simulink model "eCS_Old_Algo_And_Tests"  (R2015b)
settings: Solver=VariableStepAuto  StartTime=0.0  StopTime=10.0  RelTol=1e-3
values from neighbouring files (symbols this model uses):
  pulsetype = 2    [Parameter_eCS_Algo.m]    (also in run_simulation.m = j; run_simulation_ActiveX.m = j)
  rotation = 0    [Parameter_eCS_Algo.m]
  SubPulseType = 1    [Parameter_eCS_Algo.m]
undefined symbols (not defined in the file or in its folder): ddv, DiscIntNeverNeededParam, ECE_45_ax, ECE_45_ay, ECE_45_time, gmw_roada_x__m_s__, gmw_roada_y__m_s__, gmw_roadtime_2kHz, Heiko_AY, Heiko_AY_time, Meldorf_HindenburgstraAcceleration_x__m_s_2_, Meldorf_HindenburgstraAcceleration_y__m_s_2_, Meldorf_HindenburgstraTime__s_, pulse_FF27, pulse_MPDB, pulse_ODB40, pulse_ODB64, pulse_USNCAP, pulsetime_FF27, pulsetime_MPDB, pulsetime_ODB40, pulsetime_ODB64, pulsetime_USNCAP, VW_416_2kHza_x_2kHz, VW_416_2kHza_y_2kHz, VW_416_2kHztime_2kHz
libraries: tllib x9, simulink x9
(part 1 of 8)
settings Model: Creator=pierre-olivier.pilot  LastModifiedBy=pierre-olivier.pilot

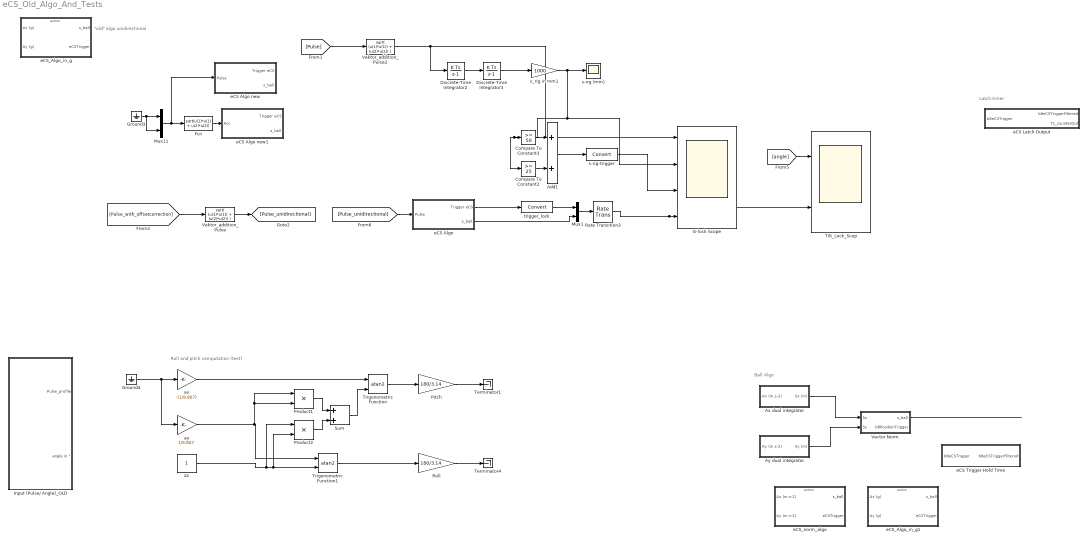
== system eCS_Old_Algo_And_Tests ==
  note: Latch timer
  note: "old" algo unidirectional
  note: Roll and pitch computation (test)
  note: Ball Algo
  Add1 : Sum
  Ax dual integrator : Subsystem  TreatAsAtomicUnit=on
  Ay dual integrator : Subsystem  TreatAsAtomicUnit=on
  Compare To Constant2 : simulink/Logic and Bit Operations/Compare To Constant  relop=>=  const=25  OutDataTypeStr=uint8
  Compare To Constant3 : simulink/Logic and Bit Operations/Compare To Constant  relop=>=  const=50  OutDataTypeStr=uint8
  Discrete-Time Integrator2 : DiscreteIntegrator  InitialConditionSetting=State (most efficient)  SampleTime=-1  ICPrevOutput=DiscIntNeverNeededParam  ICPrevScaledInput=DiscIntNeverNeededParam
  Discrete-Time Integrator3 : DiscreteIntegrator  InitialConditionSetting=State (most efficient)  SampleTime=-1  ICPrevOutput=DiscIntNeverNeededParam  ICPrevScaledInput=DiscIntNeverNeededParam
  Fcn : Fcn  Expr=sqrt(u(1)*u(1) + u(2)*u(2))
  G-lock Scope : Scope  NumInputPorts=4
  Ground3 : Ground
  Ground4 : Ground
  Input (Pulse/ Angle)_OLD : Subsystem
  Mux1 : Mux  Inputs=2
  Mux11 : Mux  Inputs=2
  Pitch : Gain  Gain=180/3.14  mask(TL_Gain){data={'date',738070.39389414352}}
      settings: CopyFcn=if exist('tl_reset_reviewflag') == 2, tl_reset_reviewflag(gcbh); end  DeleteFcn=if exist('delete_tlblock','file')==2,delete_tlblock(gcbh);end  NameChangeFcn=if exist('rename_tlblock','file')==2,rename_tlblock(gcbh);end  OpenFcn=if exist('tl_open_blockdlg','file')==2,tl_open_blockdlg(gcbh);else,open_system(gcbh,'parameter');end
      mask Help: eval(['if exist(''tl_online_help'',''file'') == 2, tl_online_help(''Topic'',''TL_Gain''),else, web([''jar:file:///'',matlabroot,''/help/toolbox/simulink/help.jar!/slref/' lower(get_param(gcbh,'Blocktype')) '.html''], ''-helpbrowser''),end'])
      mask Display: plot([0, .88, 0],[.05, .5, .93]);
  Product1 : Product  Inputs=**  RndMeth=Zero  mask(TL_Product){data={'date',738066.38423623843}}
      settings: CopyFcn=if exist('tl_reset_reviewflag') == 2, tl_reset_reviewflag(gcbh); end  DeleteFcn=if exist('delete_tlblock','file')==2,delete_tlblock(gcbh);end  NameChangeFcn=if exist('rename_tlblock','file')==2,rename_tlblock(gcbh);end  OpenFcn=if exist('tl_open_blockdlg','file')==2,tl_open_blockdlg(gcbh);else,open_system(gcbh,'parameter');end
      mask Help: eval(['if exist(''tl_online_help'',''file'') == 2, tl_online_help(''Topic'',''TL_Product''),else, web([''jar:file:///'',matlabroot,''/help/toolbox/simulink/help.jar!/slref/' lower(get_param(gcbh,'Blocktype')) '.html''], ''-helpbrowser''),end'])
      mask Display: plot([-0.1, 1.05, NaN, -0.1, 1.05],[.01, .01, NaN, .99, .99]);
  Product2 : Product  Inputs=**  RndMeth=Zero  mask(TL_Product){data={'date',738066.38423623843}}
      settings: CopyFcn=if exist('tl_reset_reviewflag') == 2, tl_reset_reviewflag(gcbh); end  DeleteFcn=if exist('delete_tlblock','file')==2,delete_tlblock(gcbh);end  NameChangeFcn=if exist('rename_tlblock','file')==2,rename_tlblock(gcbh);end  OpenFcn=if exist('tl_open_blockdlg','file')==2,tl_open_blockdlg(gcbh);else,open_system(gcbh,'parameter');end
      mask Help: eval(['if exist(''tl_online_help'',''file'') == 2, tl_online_help(''Topic'',''TL_Product''),else, web([''jar:file:///'',matlabroot,''/help/toolbox/simulink/help.jar!/slref/' lower(get_param(gcbh,'Blocktype')) '.html''], ''-helpbrowser''),end'])
      mask Display: plot([-0.1, 1.05, NaN, -0.1, 1.05],[.01, .01, NaN, .99, .99]);
  Rate Transition3 : RateTransition
  Roll : Gain  Gain=180/3.14  mask(TL_Gain){data={'date',738070.3939797685}}
      settings: CopyFcn=if exist('tl_reset_reviewflag') == 2, tl_reset_reviewflag(gcbh); end  DeleteFcn=if exist('delete_tlblock','file')==2,delete_tlblock(gcbh);end  NameChangeFcn=if exist('rename_tlblock','file')==2,rename_tlblock(gcbh);end  OpenFcn=if exist('tl_open_blockdlg','file')==2,tl_open_blockdlg(gcbh);else,open_system(gcbh,'parameter');end
      mask Help: eval(['if exist(''tl_online_help'',''file'') == 2, tl_online_help(''Topic'',''TL_Gain''),else, web([''jar:file:///'',matlabroot,''/help/toolbox/simulink/help.jar!/slref/' lower(get_param(gcbh,'Blocktype')) '.html''], ''-helpbrowser''),end'])
      mask Display: plot([0, .88, 0],[.05, .5, .93]);
  Sum : Sum  mask(TL_Sum){data={'date',738066.38487318286}}
      settings: CopyFcn=if exist('tl_reset_reviewflag') == 2, tl_reset_reviewflag(gcbh); end  DeleteFcn=if exist('delete_tlblock','file')==2,delete_tlblock(gcbh);end  NameChangeFcn=if exist('rename_tlblock','file')==2,rename_tlblock(gcbh);end  OpenFcn=if exist('tl_open_blockdlg','file')==2,tl_open_blockdlg(gcbh);else,open_system(gcbh,'parameter');end
      mask Help: eval(['if exist(''tl_online_help'',''file'') == 2, tl_online_help(''Topic'',''TL_Sum''),else, web([''jar:file:///'',matlabroot,''/help/toolbox/simulink/help.jar!/slref/' lower(get_param(gcbh,'Blocktype')) '.html''], ''-helpbrowser''),end'])
      mask Display: plot([-0.1, 1.05, NaN, -0.1, 1.05],[.01, .01, NaN, .99, .99]);
  Terminator1 : Terminator
  Terminator4 : Terminator
  Tilt_Lock_Scop : Scope  NumInputPorts=2
  Trigonometric Function : Trigonometry  Operator=atan2  mask(TL_Trigonometry){data={'date',738066.38344949076}}
      settings: CopyFcn=if exist('tl_reset_reviewflag') == 2, tl_reset_reviewflag(gcbh); end  DeleteFcn=if exist('delete_tlblock','file')==2,delete_tlblock(gcbh);end  NameChangeFcn=if exist('rename_tlblock','file')==2,rename_tlblock(gcbh);end  OpenFcn=if exist('tl_open_blockdlg','file')==2,tl_open_blockdlg(gcbh);else,open_system(gcbh,'parameter');end
      mask Help: eval(['if exist(''tl_online_help'',''file'') == 2, tl_online_help(''Topic'',''TL_Trigonometry''),else, web([''jar:file:///'',matlabroot,''/help/toolbox/simulink/help.jar!/slref/' lower(get_param(gcbh,'Blocktype')) '.html''], ''-helpbrowser''),end'])
      mask Display: plot([-0.1, 1.05, NaN, -0.1, 1.05],[.01, .01, NaN, .99, .99]);
  Trigonometric Function1 : Trigonometry  Operator=atan2  mask(TL_Trigonometry){data={'date',738066.38344949076}}
      settings: CopyFcn=if exist('tl_reset_reviewflag') == 2, tl_reset_reviewflag(gcbh); end  DeleteFcn=if exist('delete_tlblock','file')==2,delete_tlblock(gcbh);end  NameChangeFcn=if exist('rename_tlblock','file')==2,rename_tlblock(gcbh);end  OpenFcn=if exist('tl_open_blockdlg','file')==2,tl_open_blockdlg(gcbh);else,open_system(gcbh,'parameter');end
      mask Help: eval(['if exist(''tl_online_help'',''file'') == 2, tl_online_help(''Topic'',''TL_Trigonometry''),else, web([''jar:file:///'',matlabroot,''/help/toolbox/simulink/help.jar!/slref/' lower(get_param(gcbh,'Blocktype')) '.html''], ''-helpbrowser''),end'])
      mask Display: plot([-0.1, 1.05, NaN, -0.1, 1.05],[.01, .01, NaN, .99, .99]);
  Vector Norm : Subsystem  TreatAsAtomicUnit=on
  Vektor_addition_Pulse : Fcn  Expr=sqrt( (u(1)*u(1)) + (u(2)*u(2)) )
  Vektor_addition_Pulse2 : Fcn  Expr=sqrt( (u(1)*u(1)) + (u(2)*u(2)) )
  ax : Gain  Gain=-(1/9.807)  mask(TL_Gain){data={'date',738066.38476944447}}
      settings: CopyFcn=if exist('tl_reset_reviewflag') == 2, tl_reset_reviewflag(gcbh); end  DeleteFcn=if exist('delete_tlblock','file')==2,delete_tlblock(gcbh);end  NameChangeFcn=if exist('rename_tlblock','file')==2,rename_tlblock(gcbh);end  OpenFcn=if exist('tl_open_blockdlg','file')==2,tl_open_blockdlg(gcbh);else,open_system(gcbh,'parameter');end
      mask Help: eval(['if exist(''tl_online_help'',''file'') == 2, tl_online_help(''Topic'',''TL_Gain''),else, web([''jar:file:///'',matlabroot,''/help/toolbox/simulink/help.jar!/slref/' lower(get_param(gcbh,'Blocktype')) '.html''], ''-helpbrowser''),end'])
      mask Display: plot([0, .88, 0],[.05, .5, .93]);
  ay : Gain  Gain=1/9.807  mask(TL_Gain){data={'date',738066.375747037}}
      settings: CopyFcn=if exist('tl_reset_reviewflag') == 2, tl_reset_reviewflag(gcbh); end  DeleteFcn=if exist('delete_tlblock','file')==2,delete_tlblock(gcbh);end  NameChangeFcn=if exist('rename_tlblock','file')==2,rename_tlblock(gcbh);end  OpenFcn=if exist('tl_open_blockdlg','file')==2,tl_open_blockdlg(gcbh);else,open_system(gcbh,'parameter');end
      mask Help: eval(['if exist(''tl_online_help'',''file'') == 2, tl_online_help(''Topic'',''TL_Gain''),else, web([''jar:file:///'',matlabroot,''/help/toolbox/simulink/help.jar!/slref/' lower(get_param(gcbh,'Blocktype')) '.html''], ''-helpbrowser''),end'])
      mask Display: plot([0, .88, 0],[.05, .5, .93]);
  az : Constant  mask(TL_Constant){data={'date',738066.3759991898}}
      settings: CopyFcn=if exist('tl_reset_reviewflag') == 2, tl_reset_reviewflag(gcbh); end  DeleteFcn=if exist('delete_tlblock','file')==2,delete_tlblock(gcbh);end  NameChangeFcn=if exist('rename_tlblock','file')==2,rename_tlblock(gcbh);end  OpenFcn=if exist('tl_open_blockdlg','file')==2,tl_open_blockdlg(gcbh);else,open_system(gcbh,'parameter');end
      mask Help: eval(['if exist(''tl_online_help'',''file'') == 2, tl_online_help(''Topic'',''TL_Constant''),else, web([''jar:file:///'',matlabroot,''/help/toolbox/simulink/help.jar!/slref/' lower(get_param(gcbh,'Blocktype')) '.html''], ''-helpbrowser''),end'])
      mask Display: plot([-0.1, 1.05, NaN, -0.1, 1.05],[.01, .01, NaN, .99, .99]);
  eCS Algo : Subsystem
  eCS Algo new : Subsystem
  eCS Algo new1 : Subsystem
  eCS Latch Output : Subsystem  TreatAsAtomicUnit=on
  eCS Trigger Hold Time : Subsystem  TreatAsAtomicUnit=on
  eCS_Algo_in_g : Subsystem
  eCS_Algo_in_g1 : Subsystem
  eCS_norm_algo : Subsystem
  s-rig (mm) : Scope
  s-rig-trigger : DataTypeConversion
  s_rig in mm1 : Gain  Gain=1000
  trigger_lock : DataTypeConversion
  wires:
  Mux1/1 -> Rate Transition3/1
  eCS Algo/1(Trigger eCS) -> trigger_lock/1
  trigger_lock/1 -> Mux1/1
  eCS Algo/2(s_ball) -> Mux1/2
  [angle] -> Tilt_Lock_Scop/1
  Vektor_addition_Pulse/1 -> [Pulse_unidirectional]
  [Pulse_unidirectional] -> eCS Algo/1(Pulse)
  Discrete-Time Integrator2/1 -> Discrete-Time Integrator3/1
  Discrete-Time Integrator3/1 -> s_rig in mm1/1
  Vektor_addition_Pulse2/1 -> Discrete-Time Integrator2/1, G-lock Scope/1
  Compare To Constant2/1 -> Add1/2
  Compare To Constant3/1 -> Add1/1
  s_rig in mm1/1 -> G-lock Scope/2, Compare To Constant2/1, Compare To Constant3/1, s-rig (mm)/1
  Add1/1 -> s-rig-trigger/1
  s-rig-trigger/1 -> G-lock Scope/3
  [Pulse_with_offsetcorrection] -> Vektor_addition_Pulse/1
  [Pulse] -> Vektor_addition_Pulse2/1
  Rate Transition3/1 -> G-lock Scope/4, Tilt_Lock_Scop/2
  Fcn/1 -> eCS Algo new1/1(Acc)
  Mux11/1 -> eCS Algo new/1(Pulse), Fcn/1
  Ground3/1 -> Mux11/2, Mux11/1
  ay/1 -> Product1/2, Product1/1, Trigonometric Function1/1
  az/1 -> Product2/1, Product2/2, Trigonometric Function1/2
  Trigonometric Function1/1 -> Roll/1
  Product1/1 -> Sum/1
  Product2/1 -> Sum/2
  Sum/1 -> Trigonometric Function/2
  Trigonometric Function/1 -> Pitch/1
  Pitch/1 -> Terminator1/1
  Roll/1 -> Terminator4/1
  ax/1 -> Trigonometric Function/1
  Ground4/1 -> ay/1, ax/1
  ? -> Ax dual integrator/1(Ax (m.s-2))
  Vector Norm/1(s_ball) -> ?
  Ax dual integrator/1(Sx (m)) -> Vector Norm/1(Sx)
  Ay dual integrator/1(Sy (m)) -> Vector Norm/2(Sy)
  ? -> Ay dual integrator/1(Ay (m.s-2))

== system eCS_Old_Algo_And_Tests/Ax dual integrator ==
  note: sc: 1e-6
  note: [--64; 63]m.s² => [-32768 ; +32767] LSB
      | scaling : 2^-9
  note: [0 ;25]
  note: [0 ; 25]
  note: Sat [-0.0001 ; 0.0001]g.s²
      | [-10000;10000] LSB
      | scaling : 1e-8
  note: [-2 ; +2] g
      | [-32768 ; 32767] LSB
  note: [-1 : 1]
  note: sc: 1e-6
  note: x-axis : 1e-8
      | y-axis : 1e-4
      | output : 1e-4
  note: sc: 1e-3
  note: sc: 1e-3
  note: sc: 1e-3
  note: sc: 1e-4
  Ax (m.s-2) : Inport
  AddAngle : Sum  mask(TL_Sum){data={'output',{'scaling','PowerOf2/scAngle'},'date',738069.59706952551}}
      settings: CopyFcn=if exist('tl_reset_reviewflag','file')==2,tl_reset_reviewflag(gcbh);end  DeleteFcn=if exist('delete_tlblock','file')==2,delete_tlblock(gcbh);end  NameChangeFcn=if exist('rename_tlblock','file')==2,rename_tlblock(gcbh);end  OpenFcn=if exist('tl_open_blockdlg','file')==2,tl_open_blockdlg(gcbh);else,open_system(gcbh,'parameter');end
      mask Help: eval(['if exist(''tl_online_help'',''file'') == 2, tl_online_help(''Topic'',''TL_Sum''),else, web([''jar:file:///'',matlabroot,''/help/toolbox/simulink/help.jar!/slref/' lower(get_param(gcbh,'Blocktype')) '.html''], ''-helpbrowser''),end'])
      mask Display: plot([-0.1, 1.05, NaN, -0.1, 1.05],[.01, .01, NaN, .99, .99]);
  AddAx : Sum  Inputs=+--  mask(TL_Sum){data={'output',{'type','Int32','scaling','MperSecSqd_Algo/scIntegV_SI'},'date',737961.5188836921}}
      settings: CopyFcn=if exist('tl_reset_reviewflag','file')==2,tl_reset_reviewflag(gcbh);end  DeleteFcn=if exist('delete_tlblock','file')==2,delete_tlblock(gcbh);end  NameChangeFcn=if exist('rename_tlblock','file')==2,rename_tlblock(gcbh);end  OpenFcn=if exist('tl_open_blockdlg','file')==2,tl_open_blockdlg(gcbh);else,open_system(gcbh,'parameter');end
      mask Help: eval(['if exist(''tl_online_help'',''file'') == 2, tl_online_help(''Topic'',''TL_Sum''),else, web([''jar:file:///'',matlabroot,''/help/toolbox/simulink/help.jar!/slref/' lower(get_param(gcbh,'Blocktype')) '.html''], ''-helpbrowser''),end'])
      mask Display: plot([-0.1, 1.05, NaN, -0.1, 1.05],[.01, .01, NaN, .99, .99]);
  AxCalotteAngle1 : Gain  Gain=ddv('eCS_CFG/g_algo/S16_CALOTTE_ANGLE_1')  mask(TL_Gain){data={'output',{'scaling','PowerOf2/scAngle'},'gain',{'variable','eCS_CFG/g_algo/S16_CALOTTE_ANGLE_1'},'date',737958.35980387731}}
      settings: CopyFcn=if exist('tl_reset_reviewflag','file')==2,tl_reset_reviewflag(gcbh);end  DeleteFcn=if exist('delete_tlblock','file')==2,delete_tlblock(gcbh);end  NameChangeFcn=if exist('rename_tlblock','file')==2,rename_tlblock(gcbh);end  OpenFcn=if exist('tl_open_blockdlg','file')==2,tl_open_blockdlg(gcbh);else,open_system(gcbh,'parameter');end
      mask Help: eval(['if exist(''tl_online_help'',''file'') == 2, tl_online_help(''Topic'',''TL_Gain''),else, web([''jar:file:///'',matlabroot,''/help/toolbox/simulink/help.jar!/slref/' lower(get_param(gcbh,'Blocktype')) '.html''], ''-helpbrowser''),end'])
      mask Display: plot([0, .88, 0],[.05, .5, .93]);
  AxCalotteAngle2 : Gain  Gain=ddv('eCS_CFG/g_algo/S16_CALOTTE_ANGLE_2')  mask(TL_Gain){data={'output',{'scaling','PowerOf2/scAngle'},'gain',{'variable','eCS_CFG/g_algo/S16_CALOTTE_ANGLE_2'},'date',737958.35993886576}}
      settings: CopyFcn=if exist('tl_reset_reviewflag','file')==2,tl_reset_reviewflag(gcbh);end  DeleteFcn=if exist('delete_tlblock','file')==2,delete_tlblock(gcbh);end  NameChangeFcn=if exist('rename_tlblock','file')==2,rename_tlblock(gcbh);end  OpenFcn=if exist('tl_open_blockdlg','file')==2,tl_open_blockdlg(gcbh);else,open_system(gcbh,'parameter');end
      mask Help: eval(['if exist(''tl_online_help'',''file'') == 2, tl_online_help(''Topic'',''TL_Gain''),else, web([''jar:file:///'',matlabroot,''/help/toolbox/simulink/help.jar!/slref/' lower(get_param(gcbh,'Blocktype')) '.html''], ''-helpbrowser''),end'])
      mask Display: plot([0, .88, 0],[.05, .5, .93]);
  BallDamperSat : Saturate  UpperLimit=ddv('eCS_CFG/SI_Algo/BALL_DAMPER_SAT_MAX_SI')  LowerLimit=ddv('eCS_CFG/SI_Algo/BALL_DAMPER_SAT_MIN_SI')  mask(TL_Saturate){data={'output',{'type','Int32','scaling','MperSecSqd_Algo/scIntegV_SI'},'lowerlimit',{'variable','eCS_CFG/SI_Algo/BALL_DAMPER_SAT_MIN_SI'},'upperlimit',{'variable','eCS_CFG/SI_Algo/BALL_DAMPER_SAT_MAX_SI'},'date',737957.66559072922}}
      settings: CopyFcn=if exist('tl_reset_reviewflag','file')==2,tl_reset_reviewflag(gcbh);end  DeleteFcn=if exist('delete_tlblock','file')==2,delete_tlblock(gcbh);end  NameChangeFcn=if exist('rename_tlblock','file')==2,rename_tlblock(gcbh);end  OpenFcn=if exist('tl_open_blockdlg','file')==2,tl_open_blockdlg(gcbh);else,open_system(gcbh,'parameter');end
      mask Help: eval(['if exist(''tl_online_help'',''file'') == 2, tl_online_help(''Topic'',''TL_Saturate''),else, web([''jar:file:///'',matlabroot,''/help/toolbox/simulink/help.jar!/slref/' lower(get_param(gcbh,'Blocktype')) '.html''], ''-helpbrowser''),end'])
      mask Display: plot([-0.1, 1.05, NaN, -0.1, 1.05],[.01, .01, NaN, .99, .99]);
  Function : tllib/Function  data={'stepfunctionname','ComputeSx_m','date',737954.54478201387}  displayString=FUNCTION
  IntegSx : DiscreteIntegrator  SampleTime=-1  LimitOutput=on  UpperSaturationLimit=ddv('eCS_CFG/SI_Algo/BALL_POS_MAX_SI')  LowerSaturationLimit=ddv('eCS_CFG/SI_Algo/BALL_POS_MIN_SI')  ICPrevOutput=DiscIntNeverNeededParam  ICPrevScaledInput=DiscIntNeverNeededParam  mask(TL_DiscreteIntegrator){data={'output',{'scaling','MperSecSqd_Algo/scIntegS_SI'},'state',{'scaling','MperSecSqd_Algo/scIntegS_SI'},'lowerlimit',{'variable','eCS_CFG/SI_Algo/BALL_POS_MIN_SI'},'upperlimit',{'variable','eCS_CFG/SI_Algo/BALL_POS_MAX_SI'},'date',738070.37485532404}}
      settings: CopyFcn=if exist('tl_reset_reviewflag') == 2, tl_reset_reviewflag(gcbh); end  DeleteFcn=if exist('delete_tlblock','file')==2,delete_tlblock(gcbh);end  NameChangeFcn=if exist('rename_tlblock','file')==2,rename_tlblock(gcbh);end  OpenFcn=if exist('tl_open_blockdlg','file')==2,tl_open_blockdlg(gcbh);else,open_system(gcbh,'parameter');end
      mask Help: eval(['if exist(''tl_online_help'',''file'') == 2, tl_online_help(''Topic'',''TL_DiscreteIntegrator''),else, web([''jar:file:///'',matlabroot,''/help/toolbox/simulink/help.jar!/slref/' lower(get_param(gcbh,'Blocktype')) '.html''], ''-helpbrowser''),end'])
      mask Display: plot([-0.1, 1.05, NaN, -0.1, 1.05],[.01, .01, NaN, .99, .99]);
  IntegVx : DiscreteIntegrator  SampleTime=-1  ICPrevOutput=DiscIntNeverNeededParam  ICPrevScaledInput=DiscIntNeverNeededParam  mask(TL_DiscreteIntegrator){data={'output',{'scaling','MperSecSqd_Algo/scIntegV_SI'},'state',{'scaling','MperSecSqd_Algo/scIntegV_SI'},'date',737961.51929460652}}
      settings: CopyFcn=if exist('tl_reset_reviewflag') == 2, tl_reset_reviewflag(gcbh); end  DeleteFcn=if exist('delete_tlblock','file')==2,delete_tlblock(gcbh);end  NameChangeFcn=if exist('rename_tlblock','file')==2,rename_tlblock(gcbh);end  OpenFcn=if exist('tl_open_blockdlg','file')==2,tl_open_blockdlg(gcbh);else,open_system(gcbh,'parameter');end
      mask Help: eval(['if exist(''tl_online_help'',''file'') == 2, tl_online_help(''Topic'',''TL_DiscreteIntegrator''),else, web([''jar:file:///'',matlabroot,''/help/toolbox/simulink/help.jar!/slref/' lower(get_param(gcbh,'Blocktype')) '.html''], ''-helpbrowser''),end'])
      mask Display: plot([-0.1, 1.05, NaN, -0.1, 1.05],[.01, .01, NaN, .99, .99]);
  Lut_1_SI : Lookup_n-D  NumberOfTableDimensions=1  BreakpointsForDimension1=ddv('eCS_CFG/SI_Algo/AS8LUT_CALLOTE_ANGLE_1_IDX_SI')  IndexSearchMethod=Linear search  Table=ddv('eCS_CFG/SI_Algo/AS32LUT_CALLOTE_ANGLE_1_FACT_SI')  ExtrapMethod=Clip  UseLastTableValue=on  InternalRulePriority=Speed  RndMeth=Simplest  InputSameDT=on  mask(TL_Lookup1D){data={'input',{'variable','eCS_CFG/SI_Algo/AS8LUT_CALLOTE_ANGLE_1_IDX_SI'},'output',{'scaling','PowerOf2/scLutY'},'table',{'variable','eCS_CFG/SI_Algo/AS32LUT_CALLOTE_ANGLE_1_FACT_SI'},'map',{'name','CalotteAngle1_LUT_SI','class','MERGEABLE_CONST'},'date',737958.39000141202}}
      settings: CopyFcn=if exist('tl_reset_reviewflag','file')==2,tl_reset_reviewflag(gcbh);end  DeleteFcn=if exist('delete_tlblock','file')==2,delete_tlblock(gcbh);end  NameChangeFcn=if exist('rename_tlblock','file')==2,rename_tlblock(gcbh);end  OpenFcn=if exist('tl_open_blockdlg','file')==2,tl_open_blockdlg(gcbh);else,open_system(gcbh,'parameter');end
      mask Help: eval(['if exist(''tl_online_help'',''file'') == 2, tl_online_help(''Topic'',''TL_Lookup1D''),else, web([''jar:file:///'',matlabroot,''/help/toolbox/simulink/help.jar!/slref/' lower(get_param(gcbh,'Blocktype')) '.html''], ''-helpbrowser''),end'])
      mask Display: plot([-0.1, 1.05, NaN, -0.1, 1.05],[.01, .01, NaN, .99, .99]);
  Lut_2_SI : Lookup_n-D  NumberOfTableDimensions=1  BreakpointsForDimension1=ddv('eCS_CFG/SI_Algo/LUT_CALLOTE_ANGLE_2_IDX_SI')  IndexSearchMethod=Linear search  Table=ddv('eCS_CFG/SI_Algo/LUT_CALLOTE_ANGLE_2_FACT_SI')  ExtrapMethod=Clip  UseLastTableValue=on  InternalRulePriority=Speed  RndMeth=Simplest  InputSameDT=on  mask(TL_Lookup1D){data={'input',{'variable','eCS_CFG/SI_Algo/LUT_CALLOTE_ANGLE_2_IDX_SI'},'output',{'scaling','PowerOf2/scLutY'},'table',{'variable','eCS_CFG/SI_Algo/LUT_CALLOTE_ANGLE_2_FACT_SI'},'map',{'name','CalotteAngle2_LUT_SI','class','MERGEABLE_CONST'},'date',737958.39007690968}}
      settings: CopyFcn=if exist('tl_reset_reviewflag','file')==2,tl_reset_reviewflag(gcbh);end  DeleteFcn=if exist('delete_tlblock','file')==2,delete_tlblock(gcbh);end  NameChangeFcn=if exist('rename_tlblock','file')==2,rename_tlblock(gcbh);end  OpenFcn=if exist('tl_open_blockdlg','file')==2,tl_open_blockdlg(gcbh);else,open_system(gcbh,'parameter');end
      mask Help: eval(['if exist(''tl_online_help'',''file'') == 2, tl_online_help(''Topic'',''TL_Lookup1D''),else, web([''jar:file:///'',matlabroot,''/help/toolbox/simulink/help.jar!/slref/' lower(get_param(gcbh,'Blocktype')) '.html''], ''-helpbrowser''),end'])
      mask Display: plot([-0.1, 1.05, NaN, -0.1, 1.05],[.01, .01, NaN, .99, .99]);
  Scope1 : Scope
  SinAx : Trigonometry  mask(TL_Trigonometry){data={'output',{'scaling','PowerOf2/scRadian'},'date',738070.42230274307}}
      settings: CopyFcn=if exist('tl_reset_reviewflag','file')==2,tl_reset_reviewflag(gcbh);end  DeleteFcn=if exist('delete_tlblock','file')==2,delete_tlblock(gcbh);end  NameChangeFcn=if exist('rename_tlblock','file')==2,rename_tlblock(gcbh);end  OpenFcn=if exist('tl_open_blockdlg','file')==2,tl_open_blockdlg(gcbh);else,open_system(gcbh,'parameter');end
      mask Help: eval(['if exist(''tl_online_help'',''file'') == 2, tl_online_help(''Topic'',''TL_Trigonometry''),else, web([''jar:file:///'',matlabroot,''/help/toolbox/simulink/help.jar!/slref/' lower(get_param(gcbh,'Blocktype')) '.html''], ''-helpbrowser''),end'])
      mask Display: plot([-0.1, 1.05, NaN, -0.1, 1.05],[.01, .01, NaN, .99, .99]);
  ball damper : Gain  Gain=ddv('eCS_CFG/g_algo/BALL_DAMPER_COEFF')  mask(TL_Gain){data={'output',{'type','Int32','scaling','MperSecSqd_Algo/scIntegV_SI'},'gain',{'variable','eCS_CFG/g_algo/BALL_DAMPER_COEFF'},'date',737958.37810400466}}
      settings: CopyFcn=if exist('tl_reset_reviewflag','file')==2,tl_reset_reviewflag(gcbh);end  DeleteFcn=if exist('delete_tlblock','file')==2,delete_tlblock(gcbh);end  NameChangeFcn=if exist('rename_tlblock','file')==2,rename_tlblock(gcbh);end  OpenFcn=if exist('tl_open_blockdlg','file')==2,tl_open_blockdlg(gcbh);else,open_system(gcbh,'parameter');end
      mask Help: eval(['if exist(''tl_online_help'',''file'') == 2, tl_online_help(''Topic'',''TL_Gain''),else, web([''jar:file:///'',matlabroot,''/help/toolbox/simulink/help.jar!/slref/' lower(get_param(gcbh,'Blocktype')) '.html''], ''-helpbrowser''),end'])
      mask Display: plot([0, .88, 0],[.05, .5, .93]);
  g to m.s² : Gain  Gain=9.807  mask(TL_Gain){data={'logdata',{'loggingmode',1},'output',{'scaling','MperSecSqd_Algo/scAccel_SI'},'date',738036.70470343751}}
      settings: CopyFcn=if exist('tl_reset_reviewflag','file')==2,tl_reset_reviewflag(gcbh);end  DeleteFcn=if exist('delete_tlblock','file')==2,delete_tlblock(gcbh);end  NameChangeFcn=if exist('rename_tlblock','file')==2,rename_tlblock(gcbh);end  OpenFcn=if exist('tl_open_blockdlg','file')==2,tl_open_blockdlg(gcbh);else,open_system(gcbh,'parameter');end
      mask Help: eval(['if exist(''tl_online_help'',''file'') == 2, tl_online_help(''Topic'',''TL_Gain''),else, web([''jar:file:///'',matlabroot,''/help/toolbox/simulink/help.jar!/slref/' lower(get_param(gcbh,'Blocktype')) '.html''], ''-helpbrowser''),end'])
      mask Display: plot([0, .88, 0],[.05, .5, .93]);
  grad in rad1 : Gain  Gain=pi/180  mask(TL_Gain){data={'output',{'scaling','PowerOf2/scLutY'},'date',737951.6866806366}}
      settings: CopyFcn=if exist('tl_reset_reviewflag','file')==2,tl_reset_reviewflag(gcbh);end  DeleteFcn=if exist('delete_tlblock','file')==2,delete_tlblock(gcbh);end  NameChangeFcn=if exist('rename_tlblock','file')==2,rename_tlblock(gcbh);end  OpenFcn=if exist('tl_open_blockdlg','file')==2,tl_open_blockdlg(gcbh);else,open_system(gcbh,'parameter');end
      mask Help: eval(['if exist(''tl_online_help'',''file'') == 2, tl_online_help(''Topic'',''TL_Gain''),else, web([''jar:file:///'',matlabroot,''/help/toolbox/simulink/help.jar!/slref/' lower(get_param(gcbh,'Blocktype')) '.html''], ''-helpbrowser''),end'])
      mask Display: plot([0, .88, 0],[.05, .5, .93]);
  Sx (m) : Outport
  wires:
  IntegSx/1 -> Sx (m)/1, Lut_1_SI/1, Lut_2_SI/1
  ball damper/1 -> BallDamperSat/1
  AddAngle/1 -> grad in rad1/1
  AxCalotteAngle2/1 -> AddAngle/2
  Lut_2_SI/1 -> AxCalotteAngle2/1
  AxCalotteAngle1/1 -> AddAngle/1
  Lut_1_SI/1 -> AxCalotteAngle1/1
  grad in rad1/1 -> SinAx/1
  BallDamperSat/1 -> AddAx/3
  IntegVx/1 -> IntegSx/1, ball damper/1
  Ax (m.s-2)/1 -> AddAx/1
  AddAx/1 -> Scope1/1, IntegVx/1  "a-ref"
  SinAx/1 -> g to m.s²/1
  g to m.s²/1 -> AddAx/2

== system eCS_Old_Algo_And_Tests/Ay dual integrator ==
  note: sc: 1e-4
  note: sc: 1e-3
  note: sc: 1e-3
  note: sc: 1e-3
  note: x-axis : 1e-8
      | y-axis : 1e-4
      | output : 1e-4
  note: sc: 1e-6
  note: [-1 : 1]
  note: [-2 ; +2] g
      | [-32768 ; 32767] LSB
  note: Sat [-0.0001 ; 0.0001]g.s²
      | [-10000;10000] LSB
      | scaling : 1e-8
  note: [0 ; 25]
  note: [0 ;25]
  note: [--64; 63]m.s² => [-32768 ; +32767] LSB
      | scaling : 2^-9
  note: sc: 1e-6
  Ay (m.s-2) : Inport
  AddAngle : Sum  mask(TL_Sum){data={'output',{'scaling','PowerOf2/scAngle'},'date',737951.68910436344}}
      settings: CopyFcn=if exist('tl_reset_reviewflag','file')==2,tl_reset_reviewflag(gcbh);end  DeleteFcn=if exist('delete_tlblock','file')==2,delete_tlblock(gcbh);end  NameChangeFcn=if exist('rename_tlblock','file')==2,rename_tlblock(gcbh);end  OpenFcn=if exist('tl_open_blockdlg','file')==2,tl_open_blockdlg(gcbh);else,open_system(gcbh,'parameter');end
      mask Help: eval(['if exist(''tl_online_help'',''file'') == 2, tl_online_help(''Topic'',''TL_Sum''),else, web([''jar:file:///'',matlabroot,''/help/toolbox/simulink/help.jar!/slref/' lower(get_param(gcbh,'Blocktype')) '.html''], ''-helpbrowser''),end'])
      mask Display: plot([-0.1, 1.05, NaN, -0.1, 1.05],[.01, .01, NaN, .99, .99]);
  AddAy : Sum  Inputs=+--  mask(TL_Sum){data={'output',{'type','Int32','scaling','MperSecSqd_Algo/scIntegV_SI'},'date',738036.68940328702}}
      settings: CopyFcn=if exist('tl_reset_reviewflag','file')==2,tl_reset_reviewflag(gcbh);end  DeleteFcn=if exist('delete_tlblock','file')==2,delete_tlblock(gcbh);end  NameChangeFcn=if exist('rename_tlblock','file')==2,rename_tlblock(gcbh);end  OpenFcn=if exist('tl_open_blockdlg','file')==2,tl_open_blockdlg(gcbh);else,open_system(gcbh,'parameter');end
      mask Help: eval(['if exist(''tl_online_help'',''file'') == 2, tl_online_help(''Topic'',''TL_Sum''),else, web([''jar:file:///'',matlabroot,''/help/toolbox/simulink/help.jar!/slref/' lower(get_param(gcbh,'Blocktype')) '.html''], ''-helpbrowser''),end'])
      mask Display: plot([-0.1, 1.05, NaN, -0.1, 1.05],[.01, .01, NaN, .99, .99]);
  AyCalotteAngle1 : Gain  Gain=ddv('eCS_CFG/g_algo/S16_CALOTTE_ANGLE_1')  mask(TL_Gain){data={'output',{'scaling','PowerOf2/scAngle'},'gain',{'variable','eCS_CFG/g_algo/S16_CALOTTE_ANGLE_1'},'date',737958.36027694447}}
      settings: CopyFcn=if exist('tl_reset_reviewflag','file')==2,tl_reset_reviewflag(gcbh);end  DeleteFcn=if exist('delete_tlblock','file')==2,delete_tlblock(gcbh);end  NameChangeFcn=if exist('rename_tlblock','file')==2,rename_tlblock(gcbh);end  OpenFcn=if exist('tl_open_blockdlg','file')==2,tl_open_blockdlg(gcbh);else,open_system(gcbh,'parameter');end
      mask Help: eval(['if exist(''tl_online_help'',''file'') == 2, tl_online_help(''Topic'',''TL_Gain''),else, web([''jar:file:///'',matlabroot,''/help/toolbox/simulink/help.jar!/slref/' lower(get_param(gcbh,'Blocktype')) '.html''], ''-helpbrowser''),end'])
      mask Display: plot([0, .88, 0],[.05, .5, .93]);
  AyCalotteAngle2 : Gain  Gain=ddv('eCS_CFG/g_algo/S16_CALOTTE_ANGLE_2')  mask(TL_Gain){data={'output',{'scaling','PowerOf2/scAngle'},'gain',{'variable','eCS_CFG/g_algo/S16_CALOTTE_ANGLE_2'},'date',737958.36034565978}}
      settings: CopyFcn=if exist('tl_reset_reviewflag','file')==2,tl_reset_reviewflag(gcbh);end  DeleteFcn=if exist('delete_tlblock','file')==2,delete_tlblock(gcbh);end  NameChangeFcn=if exist('rename_tlblock','file')==2,rename_tlblock(gcbh);end  OpenFcn=if exist('tl_open_blockdlg','file')==2,tl_open_blockdlg(gcbh);else,open_system(gcbh,'parameter');end
      mask Help: eval(['if exist(''tl_online_help'',''file'') == 2, tl_online_help(''Topic'',''TL_Gain''),else, web([''jar:file:///'',matlabroot,''/help/toolbox/simulink/help.jar!/slref/' lower(get_param(gcbh,'Blocktype')) '.html''], ''-helpbrowser''),end'])
      mask Display: plot([0, .88, 0],[.05, .5, .93]);
  BallDamperSat : Saturate  UpperLimit=ddv('eCS_CFG/SI_Algo/BALL_DAMPER_SAT_MAX_SI')  LowerLimit=ddv('eCS_CFG/SI_Algo/BALL_DAMPER_SAT_MIN_SI')  mask(TL_Saturate){data={'output',{'type','Int32','scaling','MperSecSqd_Algo/scIntegV_SI'},'lowerlimit',{'variable','eCS_CFG/SI_Algo/BALL_DAMPER_SAT_MIN_SI'},'upperlimit',{'variable','eCS_CFG/SI_Algo/BALL_DAMPER_SAT_MAX_SI'},'date',737957.66570109956}}
      settings: CopyFcn=if exist('tl_reset_reviewflag','file')==2,tl_reset_reviewflag(gcbh);end  DeleteFcn=if exist('delete_tlblock','file')==2,delete_tlblock(gcbh);end  NameChangeFcn=if exist('rename_tlblock','file')==2,rename_tlblock(gcbh);end  OpenFcn=if exist('tl_open_blockdlg','file')==2,tl_open_blockdlg(gcbh);else,open_system(gcbh,'parameter');end
      mask Help: eval(['if exist(''tl_online_help'',''file'') == 2, tl_online_help(''Topic'',''TL_Saturate''),else, web([''jar:file:///'',matlabroot,''/help/toolbox/simulink/help.jar!/slref/' lower(get_param(gcbh,'Blocktype')) '.html''], ''-helpbrowser''),end'])
      mask Display: plot([-0.1, 1.05, NaN, -0.1, 1.05],[.01, .01, NaN, .99, .99]);
  Function : tllib/Function  data={'stepfunctionname','ComputeSy_m','date',737957.66316383099}  displayString=FUNCTION
  IntegSy : DiscreteIntegrator  SampleTime=-1  LimitOutput=on  UpperSaturationLimit=ddv('eCS_CFG/SI_Algo/BALL_POS_MAX_SI')  LowerSaturationLimit=ddv('eCS_CFG/SI_Algo/BALL_POS_MIN_SI')  ICPrevOutput=DiscIntNeverNeededParam  ICPrevScaledInput=DiscIntNeverNeededParam  mask(TL_DiscreteIntegrator){data={'output',{'scaling','MperSecSqd_Algo/scIntegS_SI'},'state',{'scaling','MperSecSqd_Algo/scIntegS_SI'},'lowerlimit',{'variable','eCS_CFG/SI_Algo/BALL_POS_MIN_SI'},'upperlimit',{'variable','eCS_CFG/SI_Algo/BALL_POS_MAX_SI'},'date',738070.37508417829}}
      settings: CopyFcn=if exist('tl_reset_reviewflag') == 2, tl_reset_reviewflag(gcbh); end  DeleteFcn=if exist('delete_tlblock','file')==2,delete_tlblock(gcbh);end  NameChangeFcn=if exist('rename_tlblock','file')==2,rename_tlblock(gcbh);end  OpenFcn=if exist('tl_open_blockdlg','file')==2,tl_open_blockdlg(gcbh);else,open_system(gcbh,'parameter');end
      mask Help: eval(['if exist(''tl_online_help'',''file'') == 2, tl_online_help(''Topic'',''TL_DiscreteIntegrator''),else, web([''jar:file:///'',matlabroot,''/help/toolbox/simulink/help.jar!/slref/' lower(get_param(gcbh,'Blocktype')) '.html''], ''-helpbrowser''),end'])
      mask Display: plot([-0.1, 1.05, NaN, -0.1, 1.05],[.01, .01, NaN, .99, .99]);
  IntegVy : DiscreteIntegrator  SampleTime=-1  ICPrevOutput=DiscIntNeverNeededParam  ICPrevScaledInput=DiscIntNeverNeededParam  mask(TL_DiscreteIntegrator){data={'output',{'scaling','MperSecSqd_Algo/scIntegV_SI'},'state',{'scaling','MperSecSqd_Algo/scIntegV_SI'},'date',737961.52197425929}}
      settings: CopyFcn=if exist('tl_reset_reviewflag') == 2, tl_reset_reviewflag(gcbh); end  DeleteFcn=if exist('delete_tlblock','file')==2,delete_tlblock(gcbh);end  NameChangeFcn=if exist('rename_tlblock','file')==2,rename_tlblock(gcbh);end  OpenFcn=if exist('tl_open_blockdlg','file')==2,tl_open_blockdlg(gcbh);else,open_system(gcbh,'parameter');end
      mask Help: eval(['if exist(''tl_online_help'',''file'') == 2, tl_online_help(''Topic'',''TL_DiscreteIntegrator''),else, web([''jar:file:///'',matlabroot,''/help/toolbox/simulink/help.jar!/slref/' lower(get_param(gcbh,'Blocktype')) '.html''], ''-helpbrowser''),end'])
      mask Display: plot([-0.1, 1.05, NaN, -0.1, 1.05],[.01, .01, NaN, .99, .99]);
  Lut_1_SI : Lookup_n-D  NumberOfTableDimensions=1  BreakpointsForDimension1=ddv('eCS_CFG/SI_Algo/AS8LUT_CALLOTE_ANGLE_1_IDX_SI')  IndexSearchMethod=Linear search  Table=ddv('eCS_CFG/SI_Algo/AS32LUT_CALLOTE_ANGLE_1_FACT_SI')  ExtrapMethod=Clip  UseLastTableValue=on  InternalRulePriority=Speed  RndMeth=Simplest  InputSameDT=on  mask(TL_Lookup1D){data={'input',{'variable','eCS_CFG/SI_Algo/AS8LUT_CALLOTE_ANGLE_1_IDX_SI'},'output',{'scaling','PowerOf2/scLutY'},'table',{'variable','eCS_CFG/SI_Algo/AS32LUT_CALLOTE_ANGLE_1_FACT_SI'},'map',{'name','CalotteAngle1_LUT_SI','class','MERGEABLE_CONST'},'date',737958.39018503472}}
      settings: CopyFcn=if exist('tl_reset_reviewflag','file')==2,tl_reset_reviewflag(gcbh);end  DeleteFcn=if exist('delete_tlblock','file')==2,delete_tlblock(gcbh);end  NameChangeFcn=if exist('rename_tlblock','file')==2,rename_tlblock(gcbh);end  OpenFcn=if exist('tl_open_blockdlg','file')==2,tl_open_blockdlg(gcbh);else,open_system(gcbh,'parameter');end
      mask Help: eval(['if exist(''tl_online_help'',''file'') == 2, tl_online_help(''Topic'',''TL_Lookup1D''),else, web([''jar:file:///'',matlabroot,''/help/toolbox/simulink/help.jar!/slref/' lower(get_param(gcbh,'Blocktype')) '.html''], ''-helpbrowser''),end'])
      mask Display: plot([-0.1, 1.05, NaN, -0.1, 1.05],[.01, .01, NaN, .99, .99]);
  Lut_2_SI : Lookup_n-D  NumberOfTableDimensions=1  BreakpointsForDimension1=ddv('eCS_CFG/SI_Algo/LUT_CALLOTE_ANGLE_2_IDX_SI')  IndexSearchMethod=Linear search  Table=ddv('eCS_CFG/SI_Algo/LUT_CALLOTE_ANGLE_2_FACT_SI')  ExtrapMethod=Clip  UseLastTableValue=on  InternalRulePriority=Speed  RndMeth=Simplest  InputSameDT=on  mask(TL_Lookup1D){data={'input',{'variable','eCS_CFG/SI_Algo/LUT_CALLOTE_ANGLE_2_IDX_SI'},'output',{'scaling','PowerOf2/scLutY'},'table',{'variable','eCS_CFG/SI_Algo/LUT_CALLOTE_ANGLE_2_FACT_SI'},'map',{'name','CalotteAngle2_LUT_SI','class','MERGEABLE_CONST'},'date',737958.39026763884}}
      settings: CopyFcn=if exist('tl_reset_reviewflag','file')==2,tl_reset_reviewflag(gcbh);end  DeleteFcn=if exist('delete_tlblock','file')==2,delete_tlblock(gcbh);end  NameChangeFcn=if exist('rename_tlblock','file')==2,rename_tlblock(gcbh);end  OpenFcn=if exist('tl_open_blockdlg','file')==2,tl_open_blockdlg(gcbh);else,open_system(gcbh,'parameter');end
      mask Help: eval(['if exist(''tl_online_help'',''file'') == 2, tl_online_help(''Topic'',''TL_Lookup1D''),else, web([''jar:file:///'',matlabroot,''/help/toolbox/simulink/help.jar!/slref/' lower(get_param(gcbh,'Blocktype')) '.html''], ''-helpbrowser''),end'])
      mask Display: plot([-0.1, 1.05, NaN, -0.1, 1.05],[.01, .01, NaN, .99, .99]);
  Scope1 : Scope
  SinAy : Trigonometry  mask(TL_Trigonometry){data={'output',{'scaling','PowerOf2/scRadian'},'date',738036.69720550929}}
      settings: CopyFcn=if exist('tl_reset_reviewflag','file')==2,tl_reset_reviewflag(gcbh);end  DeleteFcn=if exist('delete_tlblock','file')==2,delete_tlblock(gcbh);end  NameChangeFcn=if exist('rename_tlblock','file')==2,rename_tlblock(gcbh);end  OpenFcn=if exist('tl_open_blockdlg','file')==2,tl_open_blockdlg(gcbh);else,open_system(gcbh,'parameter');end
      mask Help: eval(['if exist(''tl_online_help'',''file'') == 2, tl_online_help(''Topic'',''TL_Trigonometry''),else, web([''jar:file:///'',matlabroot,''/help/toolbox/simulink/help.jar!/slref/' lower(get_param(gcbh,'Blocktype')) '.html''], ''-helpbrowser''),end'])
      mask Display: plot([-0.1, 1.05, NaN, -0.1, 1.05],[.01, .01, NaN, .99, .99]);
  ball damper : Gain  Gain=ddv('eCS_CFG/g_algo/BALL_DAMPER_COEFF')  mask(TL_Gain){data={'output',{'type','Int32','scaling','MperSecSqd_Algo/scIntegV_SI'},'gain',{'variable','eCS_CFG/g_algo/BALL_DAMPER_COEFF'},'date',737954.48961925926}}
      settings: CopyFcn=if exist('tl_reset_reviewflag','file')==2,tl_reset_reviewflag(gcbh);end  DeleteFcn=if exist('delete_tlblock','file')==2,delete_tlblock(gcbh);end  NameChangeFcn=if exist('rename_tlblock','file')==2,rename_tlblock(gcbh);end  OpenFcn=if exist('tl_open_blockdlg','file')==2,tl_open_blockdlg(gcbh);else,open_system(gcbh,'parameter');end
      mask Help: eval(['if exist(''tl_online_help'',''file'') == 2, tl_online_help(''Topic'',''TL_Gain''),else, web([''jar:file:///'',matlabroot,''/help/toolbox/simulink/help.jar!/slref/' lower(get_param(gcbh,'Blocktype')) '.html''], ''-helpbrowser''),end'])
      mask Display: plot([0, .88, 0],[.05, .5, .93]);
  g to m.s² : Gain  Gain=9.807  mask(TL_Gain){data={'output',{'scaling','MperSecSqd_Algo/scAccel_SI'},'date',738070.42273535882}}
      settings: CopyFcn=if exist('tl_reset_reviewflag','file')==2,tl_reset_reviewflag(gcbh);end  DeleteFcn=if exist('delete_tlblock','file')==2,delete_tlblock(gcbh);end  NameChangeFcn=if exist('rename_tlblock','file')==2,rename_tlblock(gcbh);end  OpenFcn=if exist('tl_open_blockdlg','file')==2,tl_open_blockdlg(gcbh);else,open_system(gcbh,'parameter');end
      mask Help: eval(['if exist(''tl_online_help'',''file'') == 2, tl_online_help(''Topic'',''TL_Gain''),else, web([''jar:file:///'',matlabroot,''/help/toolbox/simulink/help.jar!/slref/' lower(get_param(gcbh,'Blocktype')) '.html''], ''-helpbrowser''),end'])
      mask Display: plot([0, .88, 0],[.05, .5, .93]);
  grad in rad1 : Gain  Gain=pi/180  mask(TL_Gain){data={'output',{'scaling','PowerOf2/scLutY'},'date',737951.6866806366}}
      settings: CopyFcn=if exist('tl_reset_reviewflag','file')==2,tl_reset_reviewflag(gcbh);end  DeleteFcn=if exist('delete_tlblock','file')==2,delete_tlblock(gcbh);end  NameChangeFcn=if exist('rename_tlblock','file')==2,rename_tlblock(gcbh);end  OpenFcn=if exist('tl_open_blockdlg','file')==2,tl_open_blockdlg(gcbh);else,open_system(gcbh,'parameter');end
      mask Help: eval(['if exist(''tl_online_help'',''file'') == 2, tl_online_help(''Topic'',''TL_Gain''),else, web([''jar:file:///'',matlabroot,''/help/toolbox/simulink/help.jar!/slref/' lower(get_param(gcbh,'Blocktype')) '.html''], ''-helpbrowser''),end'])
      mask Display: plot([0, .88, 0],[.05, .5, .93]);
  Sy (m) : Outport
  wires:
  g to m.s²/1 -> AddAy/2
  SinAy/1 -> g to m.s²/1
  AddAy/1 -> IntegVy/1, Scope1/1  "a-ref"
  Ay (m.s-2)/1 -> AddAy/1
  IntegVy/1 -> ball damper/1, IntegSy/1
  BallDamperSat/1 -> AddAy/3
  grad in rad1/1 -> SinAy/1
  Lut_1_SI/1 -> AyCalotteAngle1/1
  AyCalotteAngle1/1 -> AddAngle/1
  Lut_2_SI/1 -> AyCalotteAngle2/1
  AyCalotteAngle2/1 -> AddAngle/2
  AddAngle/1 -> grad in rad1/1
  ball damper/1 -> BallDamperSat/1
  IntegSy/1 -> Lut_2_SI/1, Lut_1_SI/1, Sy (m)/1

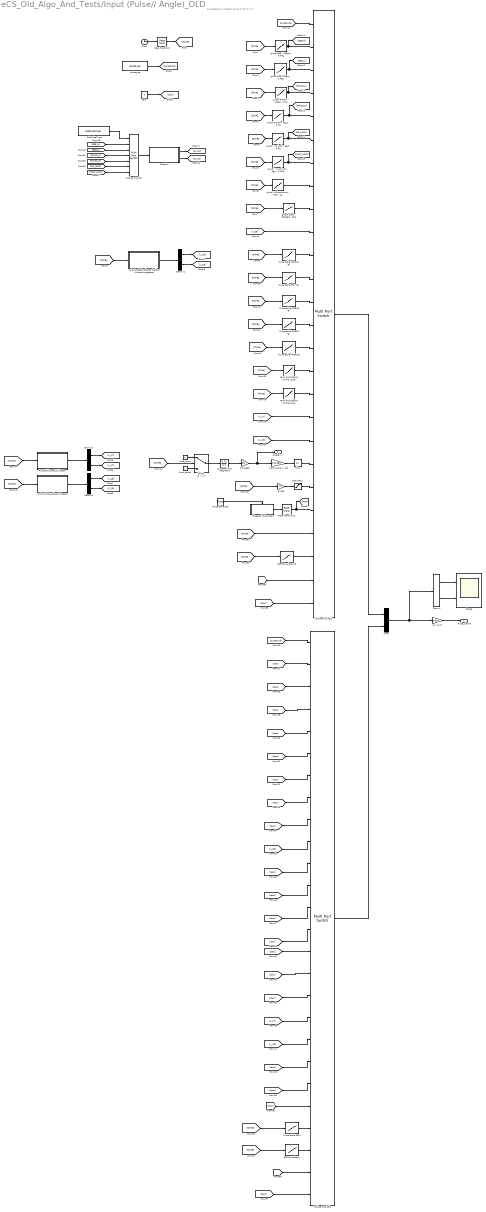
== system eCS_Old_Algo_And_Tests/Input (Pulse// Angle)_OLD ==
  note: pulse tables must begin and end with 0 !!!!!!!
  BMW QV72003-3 no-fire lower : Lookup_n-D  NumberOfTableDimensions=1  BreakpointsForDimension1=[-0.011 0.00 0.020 0.045 0.059]  Table=[0 0 11.0 11.0 0]  ExtrapMethod=Clip  UseLastTableValue=on  InternalRulePriority=Speed  RndMeth=Simplest  InputSameDT=on
  BMW QV72003-3 no-fire upper : Lookup_n-D  NumberOfTableDimensions=1  BreakpointsForDimension1=[0 0.027 0.059 0.085]  Table=[0 16.2 16.2 0]  ExtrapMethod=Clip  UseLastTableValue=on  InternalRulePriority=Speed  RndMeth=Simplest  InputSameDT=on
  Clock : Clock
  Demux{,1..3} (4 alike) : Demux  Outputs=2
  Discrete-Time Integrator4 : DiscreteIntegrator  gainval=1  InitialConditionSetting=State (most efficient)  SampleTime=-1  UpperSaturationLimit=0.3 * 9.81  LowerSaturationLimit=-0.3 * 9.81  ICPrevOutput=DiscIntNeverNeededParam  ICPrevScaledInput=DiscIntNeverNeededParam
  ECE 90 calotte 23 : Lookup  InputValues=ECE_45_time  Table=ECE_45_ax  LookUpMeth=Interpolation-Use End Values
  ECE 90 calotte y : Lookup  InputValues=ECE_45_time  Table=ECE_45_ay  LookUpMeth=Interpolation-Use End Values
  Multiport Switch : MultiPortSwitch  Inputs=6
  Multiport Switch1 : MultiPortSwitch  Inputs=24  DataPortForDefault=Additional data port
  Multiport Switch2 : MultiPortSwitch  Inputs=24  DataPortForDefault=Additional data port
  Mux1 : Mux  Inputs=2
  Puls_GWM_road_C.Morgan : Subsystem
  Puls_Kopfsteinpflaster Meldorf Hindenburgstrasse : Subsystem
  Puls_VW416_Atlas_C.Morgan : Subsystem
  Pulse Generator : DiscretePulseGenerator  PulseType=Time based  Period=0.0005  PulseWidth=5
  Pulse table ECE Y : Lookup  InputValues=Heiko_AY_time  Table=Heiko_AY  LookUpMeth=Interpolation-Use End Values
  Pulse table FF27 (g) : Lookup  InputValues=pulsetime_FF27  Table=pulse_FF27  LookUpMeth=Interpolation-Use End Values
  Pulse table MPDB (g) : Lookup  InputValues=pulsetime_MPDB  Table=pulse_MPDB  LookUpMeth=Interpolation-Use End Values
  Pulse table ODB40 (g) : Lookup  InputValues=pulsetime_ODB40  Table=pulse_ODB40  LookUpMeth=Interpolation-Use End Values
  Pulse table ODB64 (g) : Lookup  InputValues=pulsetime_ODB64  Table=pulse_ODB64  LookUpMeth=Interpolation-Use End Values
  Pulse table USNCAP (g) : Lookup  InputValues=pulsetime_USNCAP  Table=pulse_USNCAP  LookUpMeth=Interpolation-Use End Values
  Rate Transition : RateTransition
  Rate Transition2 : RateTransition
  Rotation : Subsystem
  Saturation : Saturate  UpperLimit=5  LowerLimit=0
  Scope : Scope  NumInputPorts=2
  Sin2 : Trigonometry
  SubPulseType : Constant  Value=SubPulseType
  Switch : Switch  Criteria=u2 > Threshold  Threshold=2.5
  Triggered Subsystem : Subsystem  TreatAsAtomicUnit=on
  crash angle in rad : Gain  Gain=2*pi/360
  g in m/s² : Gain  Gain=9.807
  "g-lock \" must lock\" - 6g/s - 0.45g" : Lookup_n-D  NumberOfTableDimensions=1  BreakpointsForDimension1=[0 0.075 0.3 0.4]  Table=[0 0.45 0.45 0]  ExtrapMethod=Clip  UseLastTableValue=on  InternalRulePriority=Speed  RndMeth=Simplest  InputSameDT=on
  "g-lock \" no lock\" - 6g/s - 0.3g" : Lookup_n-D  NumberOfTableDimensions=1  BreakpointsForDimension1=[0 0.050 0.5 0.6]  Table=[0 0.3 0.3 0]  ExtrapMethod=Clip  UseLastTableValue=on  InternalRulePriority=Speed  RndMeth=Simplest  InputSameDT=on
  g-lock Crash - 2000g/s - 30g : Lookup_n-D  NumberOfTableDimensions=1  BreakpointsForDimension1=[0 0.015 0.055 0.08]  Table=[0 30 30 0]  ExtrapMethod=Clip  UseLastTableValue=on  InternalRulePriority=Speed  RndMeth=Simplest  InputSameDT=on
  g-lock ECE - 150g/s - 0.45g : Lookup_n-D  NumberOfTableDimensions=1  BreakpointsForDimension1=[0 0.003 0.3 0.4]  Table=[0 0.45 0.45 0]  ExtrapMethod=Clip  UseLastTableValue=on  InternalRulePriority=Speed  RndMeth=Simplest  InputSameDT=on
  g-lock ECE - 25g/s - 0.45g : Lookup_n-D  NumberOfTableDimensions=1  BreakpointsForDimension1=[0 0.018 0.3 0.4]  Table=[0 0.45 0.45 0]  ExtrapMethod=Clip  UseLastTableValue=on  InternalRulePriority=Speed  RndMeth=Simplest  InputSameDT=on
  g-lock FMVSS  - 16g/s - 0,7g : Lookup_n-D  NumberOfTableDimensions=1  BreakpointsForDimension1=[0 0.04375 0.3 0.4]  Table=[0 0.7 0.7 0]  ExtrapMethod=Clip  UseLastTableValue=on  InternalRulePriority=Speed  RndMeth=Simplest  InputSameDT=on
  g-lock FMVSS - 70g/s - 0.7g : Lookup_n-D  NumberOfTableDimensions=1  BreakpointsForDimension1=[0 0.01 0.3 0.4]  Table=[0 0.7 0.7 0]  ExtrapMethod=Clip  UseLastTableValue=on  InternalRulePriority=Speed  RndMeth=Simplest  InputSameDT=on
  g-lock Vollbremsung - 4g/s - 1g : Lookup_n-D  NumberOfTableDimensions=1  BreakpointsForDimension1=[0 0.25 0.9745 1.2]  Table=[0 1 1 0]  ExtrapMethod=Clip  UseLastTableValue=on  InternalRulePriority=Speed  RndMeth=Simplest  InputSameDT=on
  g_rate : Gain  Gain=5
  pulsetype : Constant  Value=pulsetype
  tilt speed : Gain  Gain=10
  time_const : Constant  Value=-1
  time_const1 : Constant
  zero : Constant  Value=0
  "Pulse_profile " : Outport
  angle in ° : Outport  Port=2
  wires:
  crash angle in rad/1 -> Sin2/1
  tilt speed/1 -> angle in °/1, crash angle in rad/1
  time_const1/1 -> Switch/3
  time_const/1 -> Switch/1
  Switch/1 -> Discrete-Time Integrator4/1
  Discrete-Time Integrator4/1 -> tilt speed/1
  g_rate/1 -> Saturation/1
  Mux1/1 -> Demux/1, g in m/s²/1
  g in m/s²/1 -> "Pulse_profile "/1
  g-lock ECE - 150g/s - 0.45g/1 -> Multiport Switch1/2, [ECE_H]
  g-lock FMVSS  - 16g/s - 0,7g/1 -> Multiport Switch1/4, [FMVSS_L]
  g-lock FMVSS - 70g/s - 0.7g/1 -> [FMVSS_H], Multiport Switch1/5
  "g-lock \" no lock\" - 6g/s - 0.3g"/1 -> [NO_LOCK], Multiport Switch1/6
  "g-lock \" must lock\" - 6g/s - 0.45g"/1 -> [MUST_LOCK], Multiport Switch1/7
  g-lock Vollbremsung - 4g/s - 1g/1 -> Multiport Switch1/8
  g-lock Crash - 2000g/s - 30g/1 -> Multiport Switch1/9
  Clock/1 -> Rate Transition/1
  [time] -> g-lock ECE - 150g/s - 0.45g/1
  [time] -> g-lock ECE - 25g/s - 0.45g/1
  [time] -> g-lock FMVSS  - 16g/s - 0,7g/1
  Rate Transition/1 -> [time]
  [time] -> g-lock FMVSS - 70g/s - 0.7g/1
  [time] -> "g-lock \" no lock\" - 6g/s - 0.3g"/1
  [time] -> "g-lock \" must lock\" - 6g/s - 0.45g"/1
  [time] -> g-lock Vollbremsung - 4g/s - 1g/1
  [time] -> g-lock Crash - 2000g/s - 30g/1
  [time] -> Pulse table USNCAP (g)/1
  [time] -> Switch/2
  [time] -> g_rate/1
  [time] -> Puls_Kopfsteinpflaster Meldorf Hindenburgstrasse/1(time in)
  Demux/1 -> Scope/1
  Demux/2 -> Scope/2
  pulsetype/1 -> [pulsetype]
  [pulsetype] -> Multiport Switch1/1
  [pulsetype] -> Multiport Switch2/1
  Puls_Kopfsteinpflaster Meldorf Hindenburgstrasse/1(pulse out [x,y] (g)) -> Demux1/1
  Demux1/1 -> [x_09]
  Demux1/2 -> [y_09]
  zero/1 -> [zero]
  [zero] -> Multiport Switch2/2
  Multiport Switch1/1 -> Mux1/1
  Multiport Switch2/1 -> Mux1/2
  [zero] -> Multiport Switch2/5
  [zero] -> Multiport Switch2/6
  [zero] -> Multiport Switch2/7
  [zero] -> Multiport Switch2/8
  [zero] -> Multiport Switch2/9
  [zero] -> Multiport Switch2/12
  [zero] -> Multiport Switch2/13
  [zero] -> Multiport Switch2/14
  [x_17] -> Multiport Switch1/18
  [x_09] -> Multiport Switch1/10
  Pulse table USNCAP (g)/1 -> Multiport Switch1/11
  [y_09] -> Multiport Switch2/10
  [zero] -> Multiport Switch2/11
  [y_17] -> Multiport Switch2/18
  [zero] -> Multiport Switch2/17
  [zero] -> Multiport Switch2/16
  [zero] -> Multiport Switch2/15
  [y_18] -> Multiport Switch2/19
  [zero] -> Multiport Switch2/20
  [zero] -> Multiport Switch2/21
  [time] -> Pulse table FF27 (g)/1
  Pulse table FF27 (g)/1 -> Multiport Switch1/12
  [time] -> Pulse table ODB40 (g)/1
  [time] -> Pulse table ODB64 (g)/1
  [time] -> Pulse table MPDB (g)/1
  BMW QV72003-3 no-fire lower/1 -> Multiport Switch1/17
  BMW QV72003-3 no-fire upper/1 -> Multiport Switch1/16
  Pulse table MPDB (g)/1 -> Multiport Switch1/15
  Pulse table ODB64 (g)/1 -> Multiport Switch1/14
  Pulse table ODB40 (g)/1 -> Multiport Switch1/13
  Saturation/1 -> Multiport Switch1/21
  Sin2/1 -> Multiport Switch1/20
  [x_18] -> Multiport Switch1/19
  [time] -> BMW QV72003-3 no-fire upper/1
  [time] -> BMW QV72003-3 no-fire lower/1
  Demux2/2 -> [y_17]
  Demux2/1 -> [x_17]
  Puls_GWM_road_C.Morgan/1(pulse out [x,y] (g)) -> Demux2/1
  [time] -> Puls_GWM_road_C.Morgan/1(time in)
  Puls_VW416_Atlas_C.Morgan/1(pulse out [x,y] (g)) -> Demux3/1
  Demux3/1 -> [x_18]
  Demux3/2 -> [y_18]
  [time] -> Puls_VW416_Atlas_C.Morgan/1(time in)
  Pulse Generator/1 -> Triggered Subsystem/Trigger
  Triggered Subsystem/1(Out1) -> Rate Transition2/1
  [POP] -> Multiport Switch2/22
  Rate Transition2/1 -> [POP], Multiport Switch1/22
  g-lock ECE - 25g/s - 0.45g/1 -> Multiport Switch1/3, [ECE_L]
  [time] -> Pulse table ECE Y/1
  [time] -> ECE 90 calotte 23/1
  [zero] -> Multiport Switch2/26
  [time] -> ECE 90 calotte y/1
  [zero] -> Multiport Switch2/4
  [zero] -> Multiport Switch2/3
  [time] -> Multiport Switch1/23
  ECE 90 calotte 23/1 -> Multiport Switch1/24
  Multiport Switch/1 -> Rotation/1(Generic_Pulse)
  SubPulseType/1 -> Multiport Switch/1
  [ECE_H] -> Multiport Switch/2
  [ECE_L] -> Multiport Switch/3
  [FMVSS_L] -> Multiport Switch/4
  [FMVSS_H] -> Multiport Switch/5
  [NO_LOCK] -> Multiport Switch/6
  [MUST_LOCK] -> Multiport Switch/7
  Rotation/1(ax_rot) -> [ax_rot]
  Rotation/2(ay_rot) -> [ay_rot]
  [zero] -> Multiport Switch1/26
  [ax_rot] -> Multiport Switch1/25
  ECE 90 calotte y/1 -> Multiport Switch2/24
  Pulse table ECE Y/1 -> Multiport Switch2/23
  [ay_rot] -> Multiport Switch2/25
